simulink model "lap1"  (R2022b)
settings: Solver=VariableStepAuto  StartTime=0.0  StopTime=10.0  RelTol=1e-3
settings Model: Creator=yasso  LastModifiedBy=yasso

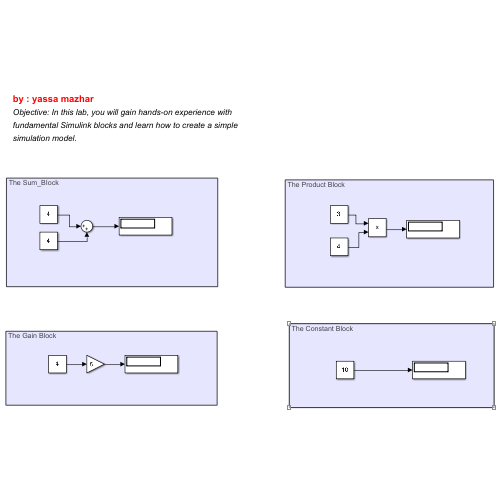
[thumbnail: Simulink's stored preview of the top-level diagram]
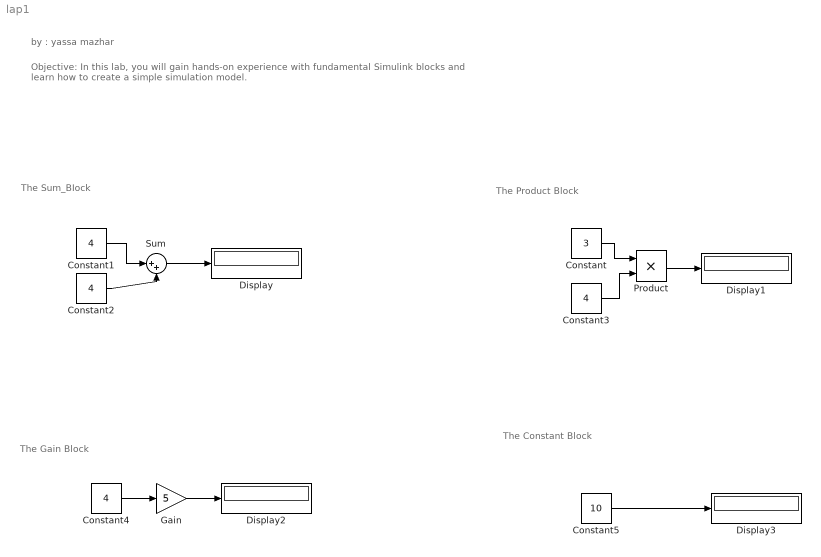
== system lap1 ==
  note: Objective: In this lab, you will gain hands-on experience with fundamental Simulink blocks and learn how to create a simple simulation model.
  note: by : yassa mazhar
  note: The Constant Block
  note: The Gain Block
  note: The Product Block
  note: The Sum_BIock
  Constant : Constant  Value=3
  Constant{1..4} (4 alike) : Constant  Value=4
  Constant5 : Constant  Value=10
  Display{,1..3} (4 alike) : Display
  Gain : Gain  Gain=5
  Product : Product
  Sum : Sum  Inputs=|++
  wires:
  Sum/1 -> Display/1
  Constant2/1 -> Sum/2
  Constant1/1 -> Sum/1
  Product/1 -> Display1/1
  Constant/1 -> Product/1
  Constant3/1 -> Product/2
  Constant4/1 -> Gain/1
  Gain/1 -> Display2/1
  Constant5/1 -> Display3/1
